simulink model "advisordemo3"  (Simulink 5.0)
settings: Solver=FixedStepDiscrete  SolverMode=SingleTasking  StartTime=0.0  StopTime=4  FixedStep=1  RelTol=1e-3  AbsTol=1e-6
libraries: fixpt_lib_4 x5
settings Model: ExecutionOrder=on  CovMetricSettings=d  Creator=andyb  LastModifiedBy=batserve  ExtModeMexFile=no_ext_comm  ExtModeTrigMode=oneshot  ExtModeArmWhenConnect=off  ExtModeAutoUpdateStatusClock=off  RTWExpressionDepthLimit=1  SaveTime=off  SaveOutput=off  LimitDataPoints=off  IntegerOverflowMsg=none  ParameterDowncastMsg=warning  ParameterOverflowMsg=warning  ParameterPrecisionLossMsg=none  RTWInlineParameters=on  ProdHWWordLengths=8,16,16,32  RTWSystemTargetFile=ert.tlc  RTWTemplateMakefile=ert_default_tmf  RTWGenerateCodeOnly=on  RTWOptions="-aCombineOutputUpdateFcns=1 -aEnforceIntegerDowncast=0 -aExtMode=0 -aExtModeTesting=0 -aFoldNonRolledExpr=1 -aForceParamTrailComments=0 -aGenFloatMathFcnCalls=\"ANSI_C\" -aGenerateASAP2=0 -aGenerateComments=1 -aGenerateErtSFunction=0 -aGenerateReport=1 -aGenerateSampleERTMain=0 -aIgnoreCustomStorageClasses=0 -aIncDataTypeInIds=1 -aIncHierarchyInIds=1 -aIncludeMdlTerminateFcn=0 -aInitFltsAndDblsToZero=0 -aInlineInvariantSignals=1 -aInlinedPrmAccess=\"Literals\" -aInsertBlockDesc=0 -aLocalBlockOutputs=1 -aMatFileLogging=0 -aMaxRTWIdLen=31 -aMultiInstanceERTCode=0 -aPrefixModelToSubsysFcnNames=1 -aPurelyIntegerCode=0 -aRTWVerbose=1 -aRollThreshold=5 -aShowEliminatedStatements=0 -aSuppressErrorStatus=1 -aZeroExternalMemoryAtStartup=0 -aZeroInternalMemoryAtStartup=0"

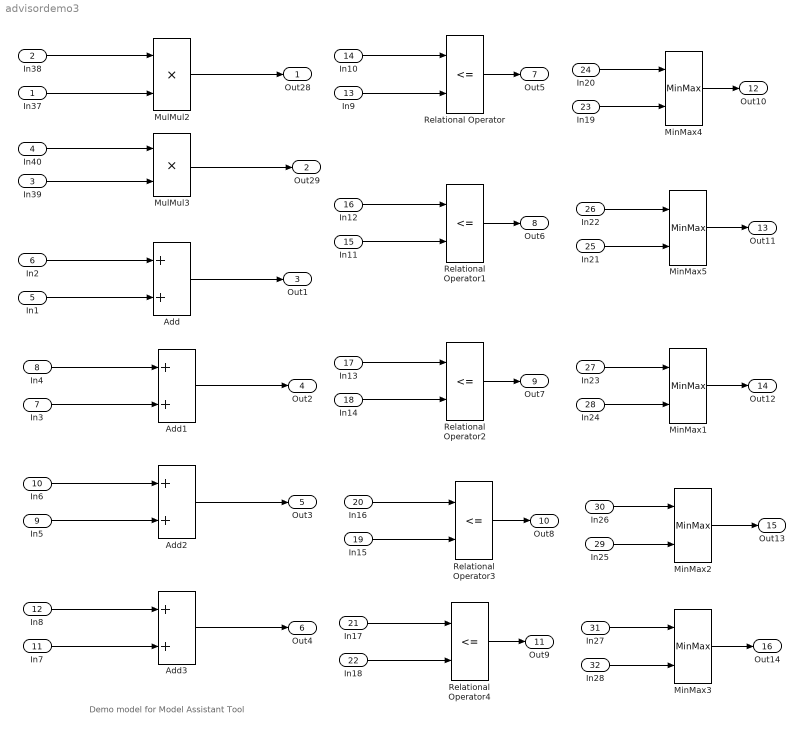
== system advisordemo3 ==
  note: Demo model for Model Assistant Tool
  In37 : Inport  PortDimensions=1  SampleTime=1  ShowAdditionalParam=on  DataType=Specify via dialog  OutScaling=1.375*2^-10  Interpolate=off
  In38 : Inport  Port=2  PortDimensions=1  SampleTime=1  ShowAdditionalParam=on  DataType=Specify via dialog  OutScaling=1.25 * 2^-10  Interpolate=off
  In39 : Inport  Port=3  PortDimensions=1  SampleTime=1  ShowAdditionalParam=on  DataType=Specify via dialog  OutScaling=2^-10  Interpolate=off
  In40 : Inport  Port=4  PortDimensions=1  SampleTime=1  ShowAdditionalParam=on  DataType=Specify via dialog  OutScaling=[2^-10 1]  Interpolate=off
  In1 : Inport  Port=5  PortDimensions=1  SampleTime=1  ShowAdditionalParam=on  DataType=Specify via dialog  OutDataType=sfix(8)  OutScaling=2^-5  Interpolate=off
  In2 : Inport  Port=6  PortDimensions=1  SampleTime=1  ShowAdditionalParam=on  DataType=Specify via dialog  OutScaling=2^-8  Interpolate=off
  In3 : Inport  Port=7  PortDimensions=1  SampleTime=1  ShowAdditionalParam=on  DataType=Specify via dialog  OutDataType=sfix(8)  OutScaling=2^-5  Interpolate=off
  In4 : Inport  Port=8  PortDimensions=1  SampleTime=1  ShowAdditionalParam=on  DataType=Specify via dialog  OutDataType=ufix(8)  OutScaling=2^-8  Interpolate=off
  In5 : Inport  Port=9  PortDimensions=1  SampleTime=1  ShowAdditionalParam=on  DataType=Specify via dialog  OutDataType=sfix(8)  OutScaling="[2^-5  6]"  Interpolate=off
  In6 : Inport  Port=10  PortDimensions=1  SampleTime=1  ShowAdditionalParam=on  DataType=Specify via dialog  OutDataType=ufix(8)  OutScaling=2^-8  Interpolate=off
  In7 : Inport  Port=11  PortDimensions=1  SampleTime=1  ShowAdditionalParam=on  DataType=Specify via dialog  OutDataType=sfix(8)  OutScaling=1.5*2^-5  Interpolate=off
  In8 : Inport  Port=12  PortDimensions=1  SampleTime=1  ShowAdditionalParam=on  DataType=Specify via dialog  OutDataType=ufix(8)  OutScaling=2^-8  Interpolate=off
  In9 : Inport  Port=13  PortDimensions=1  SampleTime=1  ShowAdditionalParam=on  DataType=Specify via dialog  OutDataType=sfix(8)  OutScaling=2^-5  Interpolate=off
  In10 : Inport  Port=14  PortDimensions=1  SampleTime=1  ShowAdditionalParam=on  DataType=Specify via dialog  OutScaling=2^-8  Interpolate=off
  In11 : Inport  Port=15  PortDimensions=1  SampleTime=1  ShowAdditionalParam=on  DataType=Specify via dialog  OutDataType=sfix(8)  OutScaling=2^-5  Interpolate=off
  In12 : Inport  Port=16  PortDimensions=1  SampleTime=1  ShowAdditionalParam=on  DataType=Specify via dialog  OutDataType=ufix(16)  OutScaling=2^-8  Interpolate=off
  In13 : Inport  Port=17  PortDimensions=1  SampleTime=1  ShowAdditionalParam=on  DataType=Specify via dialog  OutDataType=sfix(8)  OutScaling=2^-5  Interpolate=off
  In14 : Inport  Port=18  PortDimensions=1  SampleTime=1  ShowAdditionalParam=on  DataType=Specify via dialog  OutDataType=ufix(16)  OutScaling=2^-8  Interpolate=off
  In15 : Inport  Port=19  PortDimensions=1  SampleTime=1  ShowAdditionalParam=on  DataType=Specify via dialog  OutDataType=sfix(8)  OutScaling=1.125*2^-5  Interpolate=off
  In16 : Inport  Port=20  PortDimensions=1  SampleTime=1  ShowAdditionalParam=on  DataType=Specify via dialog  OutScaling=2^-8  Interpolate=off
  In17 : Inport  Port=21  PortDimensions=1  SampleTime=1  ShowAdditionalParam=on  DataType=Specify via dialog  OutDataType=sfix(8)  OutScaling=1.125*2^-5  Interpolate=off
  In18 : Inport  Port=22  PortDimensions=1  SampleTime=1  ShowAdditionalParam=on  DataType=Specify via dialog  OutScaling=2^-8  Interpolate=off
  In19 : Inport  Port=23  PortDimensions=1  SampleTime=1  ShowAdditionalParam=on  DataType=Specify via dialog  OutDataType=sfix(8)  OutScaling=2^-5  Interpolate=off
  In20 : Inport  Port=24  PortDimensions=1  SampleTime=1  ShowAdditionalParam=on  DataType=Specify via dialog  OutScaling=2^-8  Interpolate=off
  In21 : Inport  Port=25  PortDimensions=1  SampleTime=1  ShowAdditionalParam=on  DataType=Specify via dialog  OutDataType=sfix(8)  OutScaling=2^-5  Interpolate=off
  In22 : Inport  Port=26  PortDimensions=1  SampleTime=1  ShowAdditionalParam=on  DataType=Specify via dialog  OutDataType=ufix(16)  OutScaling=2^-8  Interpolate=off
  In23 : Inport  Port=27  PortDimensions=1  SampleTime=1  ShowAdditionalParam=on  DataType=Specify via dialog  OutDataType=sfix(8)  OutScaling=2^-5  Interpolate=off
  In24 : Inport  Port=28  PortDimensions=1  SampleTime=1  ShowAdditionalParam=on  DataType=Specify via dialog  OutDataType=ufix(16)  OutScaling=2^-8  Interpolate=off
  In25 : Inport  Port=29  PortDimensions=1  SampleTime=1  ShowAdditionalParam=on  DataType=Specify via dialog  OutDataType=sfix(8)  OutScaling=1.125*2^-5  Interpolate=off
  In26 : Inport  Port=30  PortDimensions=1  SampleTime=1  ShowAdditionalParam=on  DataType=Specify via dialog  OutScaling=2^-8  Interpolate=off
  In27 : Inport  Port=31  PortDimensions=1  SampleTime=1  ShowAdditionalParam=on  DataType=Specify via dialog  OutDataType=sfix(8)  OutScaling=1.125*2^-5  Interpolate=off
  In28 : Inport  Port=32  PortDimensions=1  SampleTime=1  ShowAdditionalParam=on  DataType=Specify via dialog  OutScaling=2^-8  Interpolate=off
  Add : Sum  ShowAdditionalParam=on  OutDataTypeMode=Specify via dialog  OutScaling=2^-10
  Add1 : Sum  ShowAdditionalParam=on  OutDataTypeMode=Specify via dialog  OutDataType=ufix(16)  OutScaling=2^-10
  Add2 : Sum  ShowAdditionalParam=on  OutDataTypeMode=Specify via dialog  OutDataType=ufix(16)  OutScaling=2^-10
  Add3 : Sum  ShowAdditionalParam=on  OutDataTypeMode=Specify via dialog  OutDataType=ufix(16)  OutScaling=2^-10
  MinMax{1..5} (5 alike) : fixpt_lib_4/Math/MinMax  Function=min  Inputs=2  OutDataType=sfix(16)  OutScaling=2^-10  DoSatur=off
  MulMul2 : Product  ShowAdditionalParam=on  OutDataTypeMode=Specify via dialog  OutScaling=1.5*2^-10
  MulMul3 : Product  ShowAdditionalParam=on  OutDataTypeMode=Specify via dialog  OutScaling=2^-10
  Relational Operator{,1..4} (5 alike) : RelationalOperator  Operator=<=  ShowAdditionalParam=on  LogicOutDataTypeMode=Specify via dialog  ZeroCross=off
  Out28 : Outport
  Out29 : Outport  Port=2
  Out1 : Outport  Port=3
  Out2 : Outport  Port=4
  Out3 : Outport  Port=5
  Out4 : Outport  Port=6
  Out5 : Outport  Port=7
  Out6 : Outport  Port=8
  Out7 : Outport  Port=9
  Out8 : Outport  Port=10
  Out9 : Outport  Port=11
  Out10 : Outport  Port=12
  Out11 : Outport  Port=13
  Out12 : Outport  Port=14
  Out13 : Outport  Port=15
  Out14 : Outport  Port=16
  wires:
  In37/1 -> MulMul2/2
  MulMul2/1 -> Out28/1
  In38/1 -> MulMul2/1
  In39/1 -> MulMul3/2
  MulMul3/1 -> Out29/1
  In40/1 -> MulMul3/1
  In1/1 -> Add/2
  Add/1 -> Out1/1
  In2/1 -> Add/1
  In3/1 -> Add1/2
  Add1/1 -> Out2/1
  In4/1 -> Add1/1
  In5/1 -> Add2/2
  Add2/1 -> Out3/1
  In6/1 -> Add2/1
  In7/1 -> Add3/2
  Add3/1 -> Out4/1
  In8/1 -> Add3/1
  In9/1 -> Relational Operator/2
  Relational Operator/1 -> Out5/1
  In10/1 -> Relational Operator/1
  In11/1 -> Relational Operator1/2
  Relational Operator1/1 -> Out6/1
  In12/1 -> Relational Operator1/1
  Relational Operator2/1 -> Out7/1
  In14/1 -> Relational Operator2/2
  In13/1 -> Relational Operator2/1
  In15/1 -> Relational Operator3/2
  Relational Operator3/1 -> Out8/1
  In16/1 -> Relational Operator3/1
  Relational Operator4/1 -> Out9/1
  In17/1 -> Relational Operator4/1
  In18/1 -> Relational Operator4/2
  In19/1 -> MinMax4/2
  MinMax4/1 -> Out10/1
  In20/1 -> MinMax4/1
  In21/1 -> MinMax5/2
  MinMax5/1 -> Out11/1
  In22/1 -> MinMax5/1
  MinMax1/1 -> Out12/1
  In24/1 -> MinMax1/2
  In23/1 -> MinMax1/1
  In25/1 -> MinMax2/2
  MinMax2/1 -> Out13/1
  In26/1 -> MinMax2/1
  MinMax3/1 -> Out14/1
  In27/1 -> MinMax3/1
  In28/1 -> MinMax3/2
